simulink model "Forward_speed_model"  (R2017b)
settings: Solver=ode45  StartTime=tstart  StopTime=tstop  RelTol=1e-3  EnableMultiTasking=on
values from neighbouring files (symbols this model uses):
  d1 = double(sol.d1)    [run18.m]    (also in run18_plot.m)
  d2 = double(sol.d2)    [run18.m]    (also in run18_plot.m)
  m = 5550    [run18.m]    (also in run18_plot.m)
  nc = 7.3    [run18.m]    (also in run18_plot.m)
  tsamp = 10    [run18.m]    (also in run18_plot.m)
settings Model: ExtModeAutoUpdateStatusClock=off  Creator=christh  LastModifiedBy=henningward
settings DataIOCC: LimitDataPoints=on  SaveFormat=Array  SignalLoggingSaveFormat=ModelDataLogs
settings OptimizationCC: ExpressionDepthLimit=2147483647  InitFltsAndDblsToZero=on  LifeSpan=inf
settings DebuggingCC: UnderspecifiedInitializationDetection=Classic  MergeDetectMultiDrivingBlocksExec=none  SolverPrmCheckMsg=warning  FcnCallInpInsideContextMsg=warning  StateNameClashWarn=warning  SFUnexpectedBacktrackingDiag=warning  SFNoUnconditionalDefaultTransitionDiag=warning  SFExecutionAtInitializationDiag=none
settings HardwareCC: ProdBitPerPointer=32  ProdBitPerSizeT=32  ProdBitPerPtrDiffT=32  ProdLargestAtomicFloat=None  ProdIntDivRoundTo=Undefined  ProdEndianess=Unspecified  ProdWordSize=32  ProdHWDeviceType=32-bit Generic
settings ModelReferenceCC: PropagateSignalLabelsOutOfModel=off
settings CodeAppCC: StateflowObjectComments=on
settings GRTTargetCC: TargetLangStandard=C89/C90 (ANSI)  GeneratePreprocessorConditionals=Disable all  CombineOutputUpdateFcns=off  GRTInterface=on
settings ConfigComp: CovMetricSettings=dw  CovHtmlReporting=on  CovSaveCumulativeToWorkspaceVar=on  CovSaveSingleToWorkspaceVar=on  CovExternalEMLEnable=off

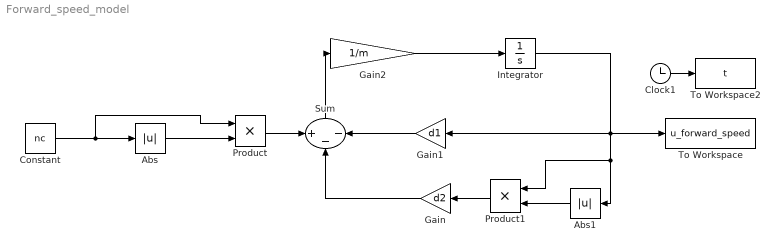
== system Forward_speed_model ==
  Abs : Abs
  Abs1 : Abs
  Clock1 : Clock
  Constant : Constant  Value=nc
  Gain : Gain  Gain=d2
  Gain1 : Gain  Gain=d1
  Gain2 : Gain  Gain=1/m
  Integrator : Integrator
  Product : Product
  Product1 : Product
  Sum : Sum  Inputs=+--
  To Workspace : ToWorkspace  VariableName=u_forward_speed  SampleTime=tsamp
  To Workspace2 : ToWorkspace  VariableName=t  SampleTime=tsamp
  wires:
  Clock1/1 -> To Workspace2/1
  Abs/1 -> Product/2
  Constant/1 -> Abs/1, Product/1
  Abs1/1 -> Product1/2
  Product1/1 -> Gain/1
  Gain1/1 -> Sum/3
  Gain/1 -> Sum/2
  Sum/1 -> Gain2/1
  Gain2/1 -> Integrator/1
  Integrator/1 -> To Workspace/1, Gain1/1, Product1/1, Abs1/1
  Product/1 -> Sum/1
